simulink library "heater_lib"  (R2020a)
settings: Solver=VariableStepAuto  StartTime=0.0  StopTime=10.0  RelTol=1e-3
settings Model: Creator=MK  LastModifiedBy=MK

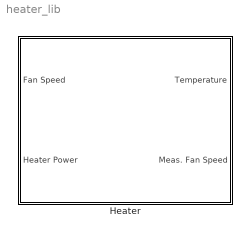
== system heater_lib ==
  Heater : Subsystem

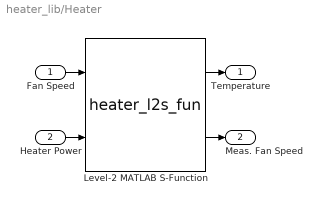
== system heater_lib/Heater ==
  Fan Speed : Inport
  Heater Power : Inport  Port=2
  Level-2 MATLAB S-Function : M-S-Function  FunctionName=heater_l2s_fun  Parameters=Ts, port
  Temperature : Outport
  Meas. Fan Speed : Outport  Port=2
  wires:
  Fan Speed/1 -> Level-2 MATLAB S-Function/1
  Level-2 MATLAB S-Function/1 -> Temperature/1
  Level-2 MATLAB S-Function/2 -> Meas. Fan Speed/1
  Heater Power/1 -> Level-2 MATLAB S-Function/2
